simulink model "HDL_source"  (R2019a)
settings: Solver=FixedStepDiscrete  StartTime=0.0  StopTime=0.1  RelTol=1e-3
PreLoadFcn:
  | load('visionhdlLaneDetectionInit.mat');
  | 
  | %Birds-Eye View Parameters:
  | T_unreal = [-0.346719845290643,-3.45626583672944e-16,-2.42608110520569e-19;-1.76272742794994,-2.62399506819665,-0.00185184300876343;1283.14845282490,1569.57420684550,1];
  | shiftleft = single([-5,-5,-5,-5,-5,-5,-5,-5,-5,-5,   -5,-4,-2,-2,-2,-2,0,0,0,1,    1,2,3,4,5,6,7,10,11,13,     15,17,20,22,26,30,33,38,42,46]);
  | shiftright = single([-20,-20,-20,-20,-20,-20,-20,-20,-20,-20,    -20,-20,-20,-21,-22,-23,-24,-24,-24,-25,    -26,-27,-28,-29,-30,-32,-33,-35,-37,-39,    -41,-45,-46,-50,-53,-57,-61,-67,-72,-78]);
StartFcn:
  | warning('off','Coder:MATLAB:polyfit_RepeatedPointsOrRescale');
  | warning('off','Coder:MATLAB:rankDeficientMatrix');
StopFcn:
  | warning('on','Coder:MATLAB:polyfit_RepeatedPointsOrRescale');
  | warning('on','Coder:MATLAB:rankDeficientMatrix');
undefined symbols (not defined in the file): gray, h1, imresize, Rec, SDTV
libraries: simulink x31, hdlsllib x19, visionhdlutilities x6, visionhdlstatistics x4, visiongeotforms x3, visionhdlio x2, visiontextngfix x2, visionhdlconversions x1, visionhdlgeotforms x1, visionhdlfilter x1, dspvision x1, visionsinks x1
(part 1 of 3)
Description:
  | Lane Detection
  | Detect lanes from streaming video.
settings Model: DataTypeOverride=Off  Creator=The MathWorks, Inc.  LastModifiedBy=timo.straessle
settings DataIOCC: SaveOutput=off  SaveTime=off  ReturnWorkspaceOutputs=off
settings OptimizationCC: BlockReduction=off  ConditionallyExecuteInputs=off  DefaultParameterBehavior=Inlined  EfficientMapNaN2IntZero=off
settings DebuggingCC: AlgebraicLoopMsg=error  SingleTaskRateTransMsg=error  ParameterPrecisionLossMsg=none  StrictBusMsg=ErrorOnBusTreatedAsVector  ArithmeticOperatorsInVariantConditions=warning
settings HardwareCC: ProdBitPerPointer=32  ProdBitPerSizeT=32  ProdBitPerPtrDiffT=32  ProdLargestAtomicFloat=None  ProdIntDivRoundTo=Undefined  ProdEndianess=Unspecified  ProdWordSize=32  ProdHWDeviceType=ASIC/FPGA->ASIC/FPGA  TargetBitPerPointer=64  TargetBitPerSizeT=64  TargetBitPerPtrDiffT=64  TargetLongLongMode=on  TargetIntDivRoundTo=Zero  TargetEndianess=LittleEndian  TargetWordSize=64  TargetHWDeviceType=MATLAB Host  ProdEqTarget=off
settings SFSimCC: SimUseLocalCustomCode=off
settings RTWCC: TLCOptions=-axpcCPUClockPoll=0
settings CodeAppCC: MaxIdLength=128
settings GRTTargetCC: TargetLangStandard=C89/C90 (ANSI)  CombineOutputUpdateFcns=off  GRTInterface=on
settings ConfigComp: CovMetricSettings=dsw  CovHtmlReporting=on  CovSaveCumulativeToWorkspaceVar=on  CovSaveSingleToWorkspaceVar=on  CovShowResultsExplorer=off  CovExternalEMLEnable=off

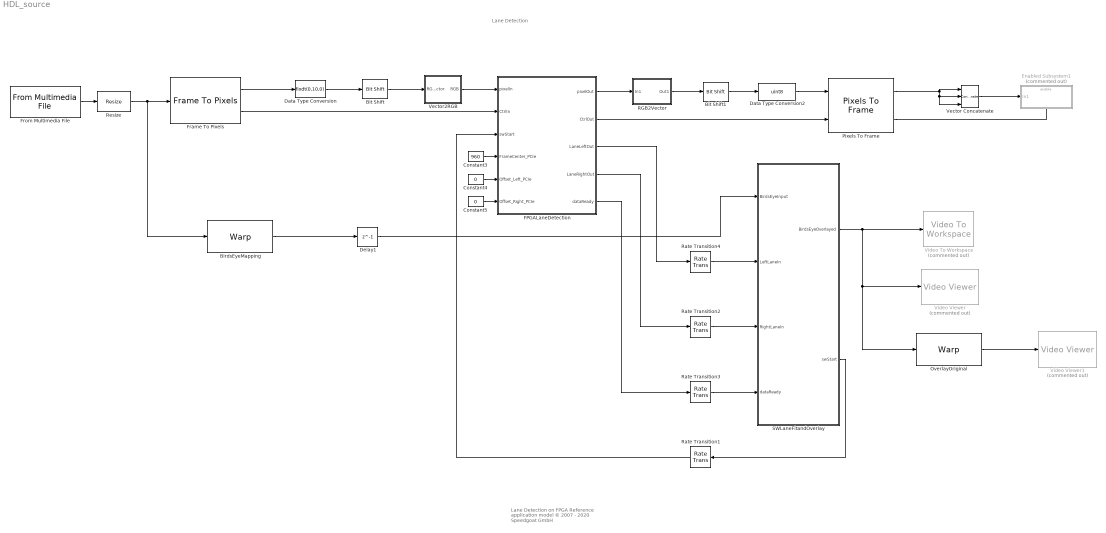
== system HDL_source ==
  note: Lane Detection
  note: Lane Detection on FPGA
      |
      | Reference application model
      | © 2007 - 2020 Speedgoat GmbH
  BirdsEyeMapping : visiongeotforms/Warp  TransformMatrixSource=Custom  TransformMatrix=T_unreal  InterpolationMethod=Bilinear  BackgroundFillValue=0  OutputImagePositionSource=Custom  OutputImagePosition=[ 1, 1, 1920, 1080 ]  ROIInputPort=off  ROIValidityOutputPort=off  SimulateUsing=Code generation
      settings: SourceProductName=Computer Vision Toolbox  SourceProductBaseCode=VP
  Bit Shift : hdlsllib/Logic and Bit Operations/Bit Shift  mode=Shift Left Logical  N=2
      settings: SourceProductName=Simulink
  Bit Shift1 : hdlsllib/Logic and Bit Operations/Bit Shift  mode=Shift Right Logical  N=2
      settings: SourceProductName=Simulink
  Constant3 : Constant  Value=960  OutDataTypeStr=fixdt(1,12,2^0,0)  SampleTime=-1
  Constant4 : Constant  Value=0  OutDataTypeStr=Inherit: Inherit via back propagation  SampleTime=-1
  Constant5 : Constant  Value=0  OutDataTypeStr=Inherit: Inherit via back propagation  SampleTime=-1
  Data Type Conversion : DataTypeConversion  OutDataTypeStr=fixdt(0,10,0)  RndMeth=Nearest
  Data Type Conversion2 : DataTypeConversion  OutDataTypeStr=uint8
  Delay1 : Delay  DelayLength=1
  Enabled Subsystem1 : Subsystem  Commented=on  TreatAsAtomicUnit=on
  FPGALaneDetection : Subsystem
  Frame To Pixels : visionhdlio/Frame To Pixels  NumComponents=3  VideoFormat=1080p  ActivePixelsPerLine=160  ActiveVideoLines=160  TotalPixelsPerLine=400  TotalVideoLines=400  StartingActiveLine=6  FrontPorch=120  SampleTime=0
      settings: SourceProductName=Vision HDL Toolbox  SourceProductBaseCode=VT
  From Multimedia File : dspvision/From Multimedia File  inputFilename=unreal.mp4  readRange=[1 Inf]  loop=on  numPlays=inf  outputStreams=Video only  videoDataType=uint8  audioDataType=int16  inheritSampleTime=off  userDefinedSampleTime=1/60  noAudioOutput=off  isIntensityVideo=off  fourcc=RGB  colorVideoFormat=One multidimensional signal  outputEOF=off  dataOrg=Column-major  audioFrameSize=1024  computeAudioFrameSize=off  outSamplingMode=Sample based
      settings: SourceProductName=DSP System Toolbox  SourceProductBaseCode=DS
  OverlayOriginal : visiongeotforms/Warp  TransformMatrixSource=Custom  TransformMatrix=inv(T_unreal)  InterpolationMethod=Bilinear  BackgroundFillValue=0  OutputImagePositionSource=Custom  OutputImagePosition=[ 1, 1, 1920, 1080 ]  ROIInputPort=off  ROIValidityOutputPort=off  SimulateUsing=Code generation
      settings: SourceProductName=Computer Vision Toolbox  SourceProductBaseCode=VP
  Pixels To Frame : visionhdlio/Pixels To Frame  NumComponents=1  VideoFormat=1080p  ActivePixelsPerLine=720  ActiveVideoLines=540  TotalPixelsPerLine=2200  TotalVideoLines=1125
      settings: SourceProductName=Vision HDL Toolbox  SourceProductBaseCode=VT
  "RGB2Vector " : Subsystem
  Rate Transition{1..4} (4 alike) : RateTransition  Deterministic=off
  Resize : visiongeotforms/Resize  specify=Number of output rows and preserve aspect ratio  rfactor=[200 150]  outCols=25  outRows=1080  outRowsCols=[25 35]  interp_method=Bilinear  antialias=on  useROI=off  roiFlag=off  roundingMode=Nearest  overflowMode=on  prodOutputMode=Binary point scaling  prodOutputWordLength=32  prodOutputFracLength=10  prodOutputSlope=2^-10  accumSlope=2^-10  outputSlope=2^-10
      settings: SourceProductName=Computer Vision Toolbox  SourceProductBaseCode=VP
  SWLaneFitandOverlay : Subsystem
  Vector Concatenate : Concatenate  NumInputs=3  Mode=Multidimensional array  ConcatenateDimension=3
  Vector2RGB : Subsystem
  Video To Workspace : visionsinks/Video To Workspace  Commented=on  VariableName=vout  NumInputs=1  DataLimit=10  DecimationFactor=1  LogFi=off  InPortLabels=R|G|B
      settings: SourceProductName=Computer Vision Toolbox  SourceProductBaseCode=VP
  Video Viewer : VideoViewer  Commented=on  colormapValue=gray(256)  FigPos=[1223 878 558 588]
  Video Viewer1 : VideoViewer  Commented=on  colormapValue=gray(256)  FigPos=[1085 664 697 473]
  wires:
  Data Type Conversion/1 -> Bit Shift/1
  Vector2RGB/1(RGB) -> FPGALaneDetection/1(pixelIn)
  Frame To Pixels/2 -> FPGALaneDetection/2(CtrlIn)
  Rate Transition1/1 -> FPGALaneDetection/3(swStart)
  FPGALaneDetection/2(CtrlOut) -> Pixels To Frame/2
  Pixels To Frame/2 -> Enabled Subsystem1/Enable
  Frame To Pixels/1 -> Data Type Conversion/1
  Bit Shift/1 -> Vector2RGB/1(RGBVector)
  OverlayOriginal/1 -> Video Viewer1/1
  Delay1/1 -> SWLaneFitandOverlay/1(BirdsEyeInput)
  FPGALaneDetection/4(LaneRightOut) -> Rate Transition2/1
  FPGALaneDetection/5(dataReady) -> Rate Transition3/1
  Rate Transition3/1 -> SWLaneFitandOverlay/4(dataReady)
  SWLaneFitandOverlay/1(BirdsEyeOverlayed) -> Video Viewer/1, OverlayOriginal/1, Video To Workspace/1
  FPGALaneDetection/3(LaneLeftOut) -> Rate Transition4/1
  SWLaneFitandOverlay/2(swStart) -> Rate Transition1/1
  BirdsEyeMapping/1 -> Delay1/1
  FPGALaneDetection/1(pixelOut) -> "RGB2Vector "/1(In1)
  Pixels To Frame/1 -> Vector Concatenate/2, Vector Concatenate/3, Vector Concatenate/1
  Vector Concatenate/1 -> Enabled Subsystem1/1(In1)
  Constant3/1 -> FPGALaneDetection/4(FrameCenter_PCIe)
  Constant4/1 -> FPGALaneDetection/5(Offset_Left_PCIe)
  Constant5/1 -> FPGALaneDetection/6(Offset_Right_PCIe)
  "RGB2Vector "/1(Out1) -> Bit Shift1/1
  Bit Shift1/1 -> Data Type Conversion2/1
  Data Type Conversion2/1 -> Pixels To Frame/1
  From Multimedia File/1 -> Resize/1
  Rate Transition4/1 -> SWLaneFitandOverlay/2(LeftLaneIn)
  Rate Transition2/1 -> SWLaneFitandOverlay/3(RightLaneIn)
  Resize/1 -> BirdsEyeMapping/1, Frame To Pixels/1

== system HDL_source/Enabled Subsystem1 ==
  In1 : Inport
  Enable : EnablePort
  To Workspace : ToWorkspace  Commented=on  VariableName=imgmat  SaveFormat=Timeseries  SampleTime=-1
  Video Viewer : VideoViewer  colormapValue=gray(256)  FigPos=[100 917 1087 696]
  wires:
  In1/1 -> To Workspace/1, Video Viewer/1

== system HDL_source/FPGALaneDetection ==
  pixelIn : Inport
  CtrlIn : Inport  Port=2
  swStart : Inport  Port=3
  FrameCenter_PCIe : Inport  Port=4
  Offset_Left_PCIe : Inport  Port=5
  Offset_Right_PCIe : Inport  Port=6
  Bit Concat : hdlsllib/Logic and Bit Operations/Bit Concat  numInputs=3
      settings: SourceProductName=Simulink
  Bit Shift1 : hdlsllib/Logic and Bit Operations/Bit Shift  mode=Shift Left Logical  N=2
      settings: SourceProductName=Simulink
  Bit Slice : hdlsllib/Logic and Bit Operations/Bit Slice  lidx=9  ridx=2
      settings: SourceProductName=Simulink  SourceProductBaseCode=SL
  Color Space Converter : visionhdlconversions/Color Space Converter  Conversion=RGB to intensity  ConversionStandard=Rec. 601 (SDTV)  ScanningStandard=1250/50/2:1  SimulateUsing=Code generation
      settings: SourceProductName=Vision HDL Toolbox  SourceProductBaseCode=VT
  Data Type Conversion1 : DataTypeConversion  OutDataTypeStr=fixdt(0,10,0)  RndMeth=Nearest
  Lane Detection Algorithm : Subsystem  TreatAsAtomicUnit=on
  "RGB2Vector " : Subsystem
  pixelOut : Outport
  CtrlOut : Outport  Port=2
  LaneLeftOut : Outport  Port=3
  LaneRightOut : Outport  Port=4
  dataReady : Outport  Port=5
  wires:
  swStart/1 -> Lane Detection Algorithm/3(swStart)
  Lane Detection Algorithm/3(LeftLane) -> LaneLeftOut/1
  Lane Detection Algorithm/4(RightLane) -> LaneRightOut/1
  Lane Detection Algorithm/5(dataReady) -> dataReady/1
  FrameCenter_PCIe/1 -> Lane Detection Algorithm/4(FrameCenter_PCIe)
  Offset_Left_PCIe/1 -> Lane Detection Algorithm/5(Offset_Left_PCIe)
  Offset_Right_PCIe/1 -> Lane Detection Algorithm/6(Offset_Right_PCIe)
  pixelIn/1 -> "RGB2Vector "/1(In1)
  "RGB2Vector "/1(Out1) -> Bit Slice/1
  CtrlIn/1 -> Color Space Converter/2
  Color Space Converter/1 -> Lane Detection Algorithm/1(YIn)
  Color Space Converter/2 -> Lane Detection Algorithm/2(CtrlIn)
  Lane Detection Algorithm/2(CtrlOut) -> CtrlOut/1
  Data Type Conversion1/1 -> Bit Shift1/1
  Bit Slice/1 -> Color Space Converter/1
  Bit Concat/1 -> pixelOut/1
  Lane Detection Algorithm/1(YOut) -> Data Type Conversion1/1
  Bit Shift1/1 -> Bit Concat/3, Bit Concat/2, Bit Concat/1

== system HDL_source/RGB2Vector  ==
  In1 : Inport
  Bit Slice2 : hdlsllib/Logic and Bit Operations/Bit Slice  lidx=9  ridx=0
      settings: SourceProductName=Simulink  SourceProductBaseCode=SL
  Out1 : Outport  VectorParamsAs1DForOutWhenUnconnected=on
  wires:
  In1/1 -> Bit Slice2/1
  Bit Slice2/1 -> Out1/1

== system HDL_source/SWLaneFitandOverlay ==
  BirdsEyeInput : Inport
  LeftLaneIn : Inport  Port=2
  RightLaneIn : Inport  Port=3
  dataReady : Inport  Port=4
  Data Type Conversion : DataTypeConversion  OutDataTypeStr=single
  Data Type Conversion1 : DataTypeConversion  OutDataTypeStr=single
  Driver : MATLAB Function  TreatAsAtomicUnit=on
  FitLanesAndOverlay : Subsystem
  Rate Transition1 : RateTransition  Deterministic=off  OutPortSampleTime=1/180
  Rate Transition2 : RateTransition  OutPortSampleTimeOpt=Inherit  OutPortSampleTime=1/60
  Signal Specification : SignalSpecification  OutDataTypeStr=boolean  Dimensions=1
  Signal Specification1 : SignalSpecification  OutDataTypeStr=boolean  Dimensions=1
  Signal Specification2 : SignalSpecification  SampleTime=1/180
  Signal Specification3 : SignalSpecification  SampleTime=1/180
  Signal Specification4 : SignalSpecification  SampleTime=1/720
  BirdsEyeOverlayed : Outport
  swStart : Outport  Port=2
  wires:
  BirdsEyeInput/1 -> FitLanesAndOverlay/1(BirdsEyeInput)
  FitLanesAndOverlay/1(OverlayOutput) -> BirdsEyeOverlayed/1
  LeftLaneIn/1 -> Signal Specification2/1
  RightLaneIn/1 -> Signal Specification3/1
  Signal Specification4/1 -> Driver/1(dataReady)
  Signal Specification/1 -> swStart/1
  Rate Transition1/1 -> FitLanesAndOverlay/Enable, Rate Transition2/1
  Rate Transition2/1 -> Signal Specification1/1
  Driver/2(process) -> Rate Transition1/1
  Signal Specification1/1 -> Driver/2(swDone)
  Driver/1(swStart) -> Signal Specification/1
  dataReady/1 -> Signal Specification4/1
  Signal Specification2/1 -> Data Type Conversion/1
  Signal Specification3/1 -> Data Type Conversion1/1
  Data Type Conversion/1 -> FitLanesAndOverlay/2(LeftLane)
  Data Type Conversion1/1 -> FitLanesAndOverlay/3(RightLane)

== system HDL_source/Vector2RGB ==
  RGBVector : Inport
  Bit Concat : hdlsllib/Logic and Bit Operations/Bit Concat  numInputs=3
      settings: SourceProductName=Simulink
  Demux : Demux  Outputs=3
  RGB : Outport  VectorParamsAs1DForOutWhenUnconnected=on
  wires:
  RGBVector/1 -> Demux/1
  Demux/1 -> Bit Concat/1
  Demux/2 -> Bit Concat/2
  Demux/3 -> Bit Concat/3
  Bit Concat/1 -> RGB/1

== system HDL_source/FPGALaneDetection/Lane Detection Algorithm ==
  YIn : Inport
  CtrlIn : Inport  Port=2
  swStart : Inport  Port=3
  FrameCenter_PCIe : Inport  Port=4
  Offset_Left_PCIe : Inport  Port=5
  Offset_Right_PCIe : Inport  Port=6
  Birds-Eye View : visionhdlgeotforms/Birds-Eye View  HomographyMatrix=T_unreal  MaxBufferSize=400000  MaxSourceLinesBuffered=200  BirdsEyeActivePixels=1920  BirdsEyeActiveLines=1080  SimulateUsing=Code generation
      settings: SourceProductName=Vision HDL Toolbox  SourceProductBaseCode=VT
  ComputeEgoLanes1 : Subsystem
  CtrlInterface1 : MATLAB Function  TreatAsAtomicUnit=on
  LaneDetection1 : Subsystem
  Signal Specification3 : SignalSpecification  Dimensions=[40 1]
  Signal Specification4 : SignalSpecification  Dimensions=[40 1]
  Signal Specification5 : SignalSpecification  OutDataTypeStr=boolean
  YOut : Outport
  CtrlOut : Outport  Port=2
  LeftLane : Outport  Port=3
  RightLane : Outport  Port=4
  dataReady : Outport  Port=5
  wires:
  Birds-Eye View/2 -> CtrlOut/1, LaneDetection1/2(ctrlIn)
  FrameCenter_PCIe/1 -> ComputeEgoLanes1/10(Frame_Center_PCIe)
  Offset_Left_PCIe/1 -> ComputeEgoLanes1/11(Offset_Left_PCIe)
  Offset_Right_PCIe/1 -> ComputeEgoLanes1/12(Offset_Right_PCIe)
  CtrlInterface1/1(LaneLeftout) -> Signal Specification3/1
  LaneDetection1/5(lane4) -> ComputeEgoLanes1/5(lane4In)
  ComputeEgoLanes1/4(start) -> CtrlInterface1/4(hwStart)
  ComputeEgoLanes1/5(done) -> CtrlInterface1/5(hwDone)
  LaneDetection1/8(lane7) -> ComputeEgoLanes1/8(lane7In)
  swStart/1 -> CtrlInterface1/6(swStart)
  LaneDetection1/7(lane6) -> ComputeEgoLanes1/7(lane6In)
  LaneDetection1/6(lane5) -> ComputeEgoLanes1/6(lane5In)
  ComputeEgoLanes1/3(enable) -> CtrlInterface1/3(enable)
  LaneDetection1/3(lane2) -> ComputeEgoLanes1/3(lane2In)
  LaneDetection1/1(enable) -> ComputeEgoLanes1/1(laneCapture)
  ComputeEgoLanes1/2(LaneRight) -> CtrlInterface1/2(LaneRightin)
  LaneDetection1/9(frameStart) -> ComputeEgoLanes1/9(frameStart)
  Signal Specification4/1 -> RightLane/1
  Signal Specification5/1 -> dataReady/1
  Signal Specification3/1 -> LeftLane/1
  CtrlInterface1/3(dataReady) -> Signal Specification5/1
  CtrlInterface1/2(LaneRightout) -> Signal Specification4/1
  ComputeEgoLanes1/1(LaneLeft) -> CtrlInterface1/1(LaneLeftin)
  LaneDetection1/4(lane3) -> ComputeEgoLanes1/4(lane3In)
  LaneDetection1/2(lane1) -> ComputeEgoLanes1/2(lane1In)
  Birds-Eye View/1 -> YOut/1, LaneDetection1/1(pixelIn)
  YIn/1 -> Birds-Eye View/1
  CtrlIn/1 -> Birds-Eye View/2

== system HDL_source/FPGALaneDetection/RGB2Vector  ==
  In1 : Inport
  Bit Slice : hdlsllib/Logic and Bit Operations/Bit Slice  lidx=29  ridx=20
      settings: SourceProductName=Simulink  SourceProductBaseCode=SL
  Bit Slice1 : hdlsllib/Logic and Bit Operations/Bit Slice  lidx=19  ridx=10
      settings: SourceProductName=Simulink  SourceProductBaseCode=SL
  Bit Slice2 : hdlsllib/Logic and Bit Operations/Bit Slice  lidx=9  ridx=0
      settings: SourceProductName=Simulink  SourceProductBaseCode=SL
  Mux : Mux  Inputs=3
  Transpose : Math  Operator=transpose  RndMeth=Zero  SaturateOnIntegerOverflow=on
  Out1 : Outport  VectorParamsAs1DForOutWhenUnconnected=on
  wires:
  In1/1 -> Bit Slice2/1, Bit Slice1/1, Bit Slice/1
  Bit Slice/1 -> Mux/1
  Bit Slice1/1 -> Mux/2
  Bit Slice2/1 -> Mux/3
  Mux/1 -> Transpose/1
  Transpose/1 -> Out1/1

== system HDL_source/SWLaneFitandOverlay/FitLanesAndOverlay ==
  BirdsEyeInput : Inport
  LeftLane : Inport  Port=2
  RightLane : Inport  Port=3
  Enable : EnablePort
  Add : Sum
  Add1 : Sum
  Constant : Constant  Value=shiftleft
  Constant1 : Constant  Value=shiftright
  FitLanes : Subsystem
  Index : Constant  Value=[1:1:40]'*27  VectorParams1D=off  OutDataTypeStr=single  SampleTime=-1
  OverlayLaneMarkings : Subsystem
  Rate Transition{,1..3} (4 alike) : RateTransition  OutPortSampleTime=1/60
  Vector Concatenate : Concatenate  Mode=Multidimensional array  ConcatenateDimension=2
  Vector Concatenate1 : Concatenate  Mode=Multidimensional array  ConcatenateDimension=2
  OverlayOutput : Outport
  wires:
  FitLanes/2(RightPolynomial) -> Rate Transition1/1
  FitLanes/1(LeftPolynomial) -> Rate Transition/1
  OverlayLaneMarkings/1(ImOut) -> OverlayOutput/1
  LeftLane/1 -> Add/2
  Rate Transition/1 -> OverlayLaneMarkings/4(LeftPolynomial)
  Rate Transition1/1 -> OverlayLaneMarkings/5(RightPolynomial)
  Vector Concatenate1/1 -> Rate Transition3/1, FitLanes/2(RightLaneCoords)
  Vector Concatenate/1 -> FitLanes/1(LeftLaneCoords), Rate Transition2/1
  BirdsEyeInput/1 -> OverlayLaneMarkings/1(ImIn)
  RightLane/1 -> Add1/2
  Index/1 -> Vector Concatenate/2, Vector Concatenate1/2
  Rate Transition2/1 -> OverlayLaneMarkings/2(LeftLaneCoords)
  Rate Transition3/1 -> OverlayLaneMarkings/3(RightLaneCoords)
  Constant/1 -> Add/1
  Add/1 -> Vector Concatenate/1
  Constant1/1 -> Add1/1
  Add1/1 -> Vector Concatenate1/1

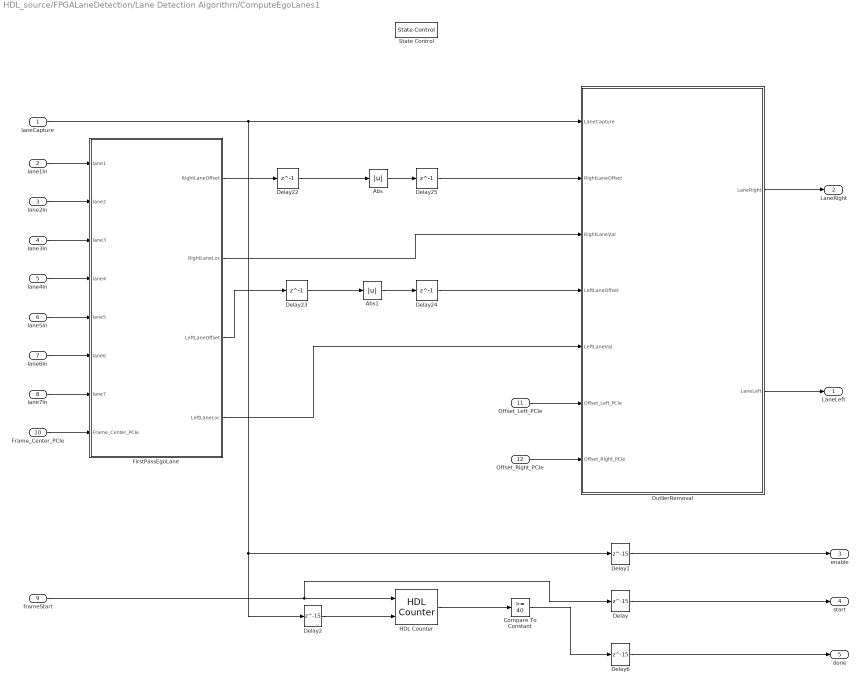
== system HDL_source/FPGALaneDetection/Lane Detection Algorithm/ComputeEgoLanes1 ==
  laneCapture : Inport
  lane1In : Inport  Port=2
  lane2In : Inport  Port=3
  lane3In : Inport  Port=4
  lane4In : Inport  Port=5
  lane5In : Inport  Port=6
  lane6In : Inport  Port=7
  lane7In : Inport  Port=8
  frameStart : Inport  Port=9
  Frame_Center_PCIe : Inport  Port=10
  Offset_Left_PCIe : Inport  Port=11
  Offset_Right_PCIe : Inport  Port=12
  Abs : Abs
  Abs1 : Abs
  Compare To Constant : simulink/Logic and Bit Operations/Compare To Constant  relop=>=  const=40  OutDataTypeStr=boolean
  Delay{,1..2,6} (4 alike) : Delay  DelayLength=15
  Delay{22..25} (4 alike) : Delay  DelayLength=1
  FirstPassEgoLane : Subsystem
  HDL Counter : hdlsllib/Sources/HDL Counter  CountType=Free running  CountInit=0  CountStep=1  CountMax=40  CountFromType=Initial value  CountFrom=0  CountResetPort=on  CountLoadPort=off  CountEnbPort=on  CountDirPort=off  CountDataType=Unsigned  CountWordLen=6  CountFracLen=0  CountSampTime=1
      settings: SourceProductName=Simulink
  OutlierRemoval : Subsystem
  State Control : StateControl  StateControl=Synchronous
  LaneLeft : Outport
  LaneRight : Outport  Port=2
  enable : Outport  Port=3
  start : Outport  Port=4
  done : Outport  Port=5
  wires:
  laneCapture/1 -> Delay1/1, Delay2/1, OutlierRemoval/1(LaneCapture)
  Abs/1 -> Delay25/1
  Abs1/1 -> Delay24/1
  lane1In/1 -> FirstPassEgoLane/1(lane1)
  lane2In/1 -> FirstPassEgoLane/2(lane2)
  lane3In/1 -> FirstPassEgoLane/3(lane3)
  lane4In/1 -> FirstPassEgoLane/4(lane4)
  lane5In/1 -> FirstPassEgoLane/5(lane5)
  lane6In/1 -> FirstPassEgoLane/6(lane6)
  lane7In/1 -> FirstPassEgoLane/7(lane7)
  FirstPassEgoLane/1(RightLaneOffset) -> Delay22/1
  FirstPassEgoLane/3(LeftLaneOffset) -> Delay23/1
  Delay22/1 -> Abs/1
  Delay23/1 -> Abs1/1
  Delay25/1 -> OutlierRemoval/2(RightLaneOffset)
  FirstPassEgoLane/2(RightLaneLoc) -> OutlierRemoval/3(RightLaneVal)
  FirstPassEgoLane/4("LeftLaneLoc ") -> OutlierRemoval/5(LeftLaneVal)
  Delay24/1 -> OutlierRemoval/4(LeftLaneOffset)
  Delay/1 -> start/1
  Delay6/1 -> done/1
  Delay1/1 -> enable/1
  OutlierRemoval/1(LaneRight) -> LaneRight/1
  OutlierRemoval/2(LaneLeft) -> LaneLeft/1
  HDL Counter/1 -> Compare To Constant/1
  frameStart/1 -> Delay/1, HDL Counter/1
  Compare To Constant/1 -> Delay6/1
  Delay2/1 -> HDL Counter/2
  Frame_Center_PCIe/1 -> FirstPassEgoLane/8(Frame_Center_PCIe)
  Offset_Left_PCIe/1 -> OutlierRemoval/6(Offset_Left_PCIe)
  Offset_Right_PCIe/1 -> OutlierRemoval/7(Offset_Right_PCIe)

== system HDL_source/FPGALaneDetection/Lane Detection Algorithm/LaneDetection1 ==
  pixelIn : Inport
  ctrlIn : Inport  Port=2
  LaneCandidateGeneration : Subsystem
  State Control : StateControl  StateControl=Synchronous
  VerticallyOrientatedFilter : visionhdlfilter/Image Filter  CoefficientsSource=Property  Coefficients=imresize(h1, 2.25)/(2.25^2)  PaddingMethod=Symmetric  PaddingValue=0  LineBufferSize=2048  SimulateUsing=Code generation  roundingMode=Round  overflowMode=on  CoeffDataTypeStr=fixdt(1,24,15)  CoeffMin=[]  CoeffMax=[]  OutputDataTypeStr=fixdt(1,24,15)  OutputMin=[]  OutputMax=[]
      settings: SourceProductName=Vision HDL Toolbox  SourceProductBaseCode=VT
  enable : Outport
  lane1 : Outport  Port=2
  lane2 : Outport  Port=3
  lane3 : Outport  Port=4
  lane4 : Outport  Port=5
  lane5 : Outport  Port=6
  lane6 : Outport  Port=7
  lane7 : Outport  Port=8
  frameStart : Outport  Port=9
  wires:
  VerticallyOrientatedFilter/2 -> LaneCandidateGeneration/2(crtlIn)
  VerticallyOrientatedFilter/1 -> LaneCandidateGeneration/1(pixelIn)
  LaneCandidateGeneration/6(lane6) -> lane6/1
  ctrlIn/1 -> VerticallyOrientatedFilter/2
  LaneCandidateGeneration/4(lane4) -> lane4/1
  LaneCandidateGeneration/3(lane3) -> lane3/1
  LaneCandidateGeneration/7(lane7) -> lane7/1
  LaneCandidateGeneration/2(lane2) -> lane2/1
  pixelIn/1 -> VerticallyOrientatedFilter/1
  LaneCandidateGeneration/8(laneCapture) -> enable/1
  LaneCandidateGeneration/5(lane5) -> lane5/1
  LaneCandidateGeneration/1(lane1) -> lane1/1
  LaneCandidateGeneration/9(frameStart) -> frameStart/1

== system HDL_source/SWLaneFitandOverlay/FitLanesAndOverlay/FitLanes ==
  LeftLaneCoords : Inport
  RightLaneCoords : Inport  Port=2
  FitLeftPolyLane : MATLAB Function  TreatAsAtomicUnit=on
  FitRightPolyLane : MATLAB Function  TreatAsAtomicUnit=on
  LeftPolynomial : Outport
  RightPolynomial : Outport  Port=2
  wires:
  FitLeftPolyLane/1(P) -> LeftPolynomial/1
  FitRightPolyLane/1(P) -> RightPolynomial/1
  LeftLaneCoords/1 -> FitLeftPolyLane/1(laneCIn)
  RightLaneCoords/1 -> FitRightPolyLane/1(laneCIn)

== system HDL_source/SWLaneFitandOverlay/FitLanesAndOverlay/OverlayLaneMarkings ==
  ImIn : Inport
  LeftLaneCoords : Inport  Port=2
  RightLaneCoords : Inport  Port=3
  LeftPolynomial : Inport  Port=4
  RightPolynomial : Inport  Port=5
  Constant{,1..3} (4 alike) : Constant  Value=ones(40,1)*30  OutDataTypeStr=single  SampleTime=-1
  Constant4 : Constant  Value=[75 1 1845 1080]  OutDataTypeStr=uint32  SampleTime=-1
  Constant5 : Constant  Value=[75 1 1845 1080]  OutDataTypeStr=uint32  SampleTime=-1
  Data Type Conversion : DataTypeConversion  OutDataTypeStr=uint32
  Data Type Conversion1 : DataTypeConversion  OutDataTypeStr=uint32
  Draw Shapes : visiontextngfix/Draw Shapes  shape=Rectangles  fill=off  lineWidth=4  fillClrSource=Specify via dialog  display=User-specified value  intensity=200  color=[83, 219, 192]  opacity=0.6  viewport=Specify region of interest via port  antialiasing=off  inType=Obsolete  imagePorts=One multidimensional signal  roundingMode=Floor  overflowMode=off  memoryMode=Specify word length  memoryWordLength=16  prodOutputMode=Binary point scaling  prodOutputWordLength=32  prodOutputFracLength=14  prodOutputSlope=2^-14  accumSlope=2^-14  memoryFracLength=15
      settings: SourceProductName=Computer Vision Toolbox
  Draw Shapes1 : visiontextngfix/Draw Shapes  shape=Rectangles  fill=off  lineWidth=4  fillClrSource=Specify via dialog  display=User-specified value  intensity=200  color=[255, 26,0]  opacity=0.6  viewport=Specify region of interest via port  antialiasing=off  inType=Obsolete  imagePorts=One multidimensional signal  roundingMode=Floor  overflowMode=off  memoryMode=Specify word length  memoryWordLength=16  prodOutputMode=Binary point scaling  prodOutputWordLength=32  prodOutputFracLength=14  prodOutputSlope=2^-14  accumSlope=2^-14  memoryFracLength=15
      settings: SourceProductName=Computer Vision Toolbox
  DrawPolynomial : MATLAB Function  TreatAsAtomicUnit=on
  OverlayPolynomialLane1 : MATLAB Function  TreatAsAtomicUnit=on
  Vector Concatenate{,1..3} (4 alike) : Concatenate  Mode=Multidimensional array  ConcatenateDimension=2
  ImOut : Outport
  wires:
  OverlayPolynomialLane1/1(Im) -> DrawPolynomial/2("Im ")
  DrawPolynomial/1(Im) -> ImOut/1
  LeftPolynomial/1 -> OverlayPolynomialLane1/1(P1)
  RightPolynomial/1 -> DrawPolynomial/1(P1)
  Constant/1 -> Vector Concatenate/2
  LeftLaneCoords/1 -> Vector Concatenate/1
  Constant1/1 -> Vector Concatenate1/2
  Vector Concatenate/1 -> Vector Concatenate1/1
  ImIn/1 -> Draw Shapes1/1
  RightLaneCoords/1 -> Vector Concatenate2/1
  Vector Concatenate1/1 -> Data Type Conversion/1
  Data Type Conversion/1 -> Draw Shapes1/2
  Draw Shapes1/1 -> Draw Shapes/1
  Vector Concatenate3/1 -> Data Type Conversion1/1
  Vector Concatenate2/1 -> Vector Concatenate3/1
  Constant3/1 -> Vector Concatenate3/2
  Constant2/1 -> Vector Concatenate2/2
  Data Type Conversion1/1 -> Draw Shapes/2
  Draw Shapes/1 -> OverlayPolynomialLane1/2("Im ")
  Constant4/1 -> Draw Shapes1/3
  Constant5/1 -> Draw Shapes/3

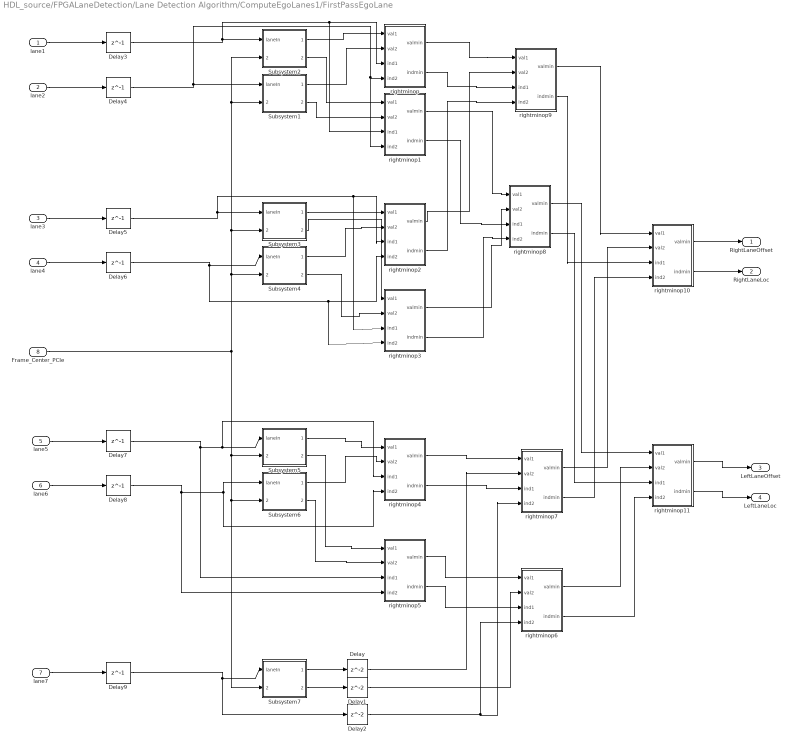
== system HDL_source/FPGALaneDetection/Lane Detection Algorithm/ComputeEgoLanes1/FirstPassEgoLane ==
  lane1 : Inport
  lane2 : Inport  Port=2
  lane3 : Inport  Port=3
  lane4 : Inport  Port=4
  lane5 : Inport  Port=5
  lane6 : Inport  Port=6
  lane7 : Inport  Port=7
  Frame_Center_PCIe : Inport  Port=8
  Delay : Delay
  Delay1 : Delay
  Delay2 : Delay
  Delay{3..9} (7 alike) : Delay  DelayLength=1
  Subsystem1 : Subsystem
  Subsystem2 : Subsystem
  Subsystem3 : Subsystem
  Subsystem4 : Subsystem
  Subsystem5 : Subsystem
  Subsystem6 : Subsystem
  Subsystem7 : Subsystem
  rightminop : Subsystem
  rightminop1 : Subsystem
  rightminop10 : Subsystem
  rightminop11 : Subsystem
  rightminop2 : Subsystem
  rightminop3 : Subsystem
  rightminop4 : Subsystem
  rightminop5 : Subsystem
  rightminop6 : Subsystem
  rightminop7 : Subsystem
  rightminop8 : Subsystem
  rightminop9 : Subsystem
  RightLaneOffset : Outport
  RightLaneLoc : Outport  Port=2
  LeftLaneOffset : Outport  Port=3
  "LeftLaneLoc " : Outport  Port=4
  wires:
  Subsystem7/2(LeftLaneVal) -> Delay1/1
  rightminop7/1(valmin) -> rightminop10/2(val2)
  rightminop9/2(indmin) -> rightminop10/3(ind1)
  rightminop3/2(indmin) -> rightminop8/4(ind2)
  rightminop7/2(indmin) -> rightminop10/4(ind2)
  Subsystem5/2(LeftLaneVal) -> rightminop5/1(val1)
  rightminop8/1(valmin) -> rightminop11/1(val1)
  Subsystem2/1(RightLaneVal) -> rightminop/1(val1)
  rightminop4/2(indmin) -> rightminop7/3(ind1)
  rightminop6/2(indmin) -> rightminop11/4(ind2)
  Subsystem1/1(RightLaneVal) -> rightminop/2(val2)
  Subsystem7/1(RightLaneVal) -> Delay/1
  Subsystem4/1(RightLaneVal) -> rightminop2/2(val2)
  rightminop5/2(indmin) -> rightminop6/3(ind1)
  rightminop6/1(valmin) -> rightminop11/2(val2)
  lane3/1 -> Delay5/1
  rightminop9/1(valmin) -> rightminop10/1(val1)
  rightminop8/2(indmin) -> rightminop11/3(ind1)
  rightminop5/1(valmin) -> rightminop6/1(val1)
  lane7/1 -> Delay9/1
  rightminop1/1(valmin) -> rightminop8/1(val1)
  rightminop11/1(valmin) -> LeftLaneOffset/1
  rightminop11/2(indmin) -> "LeftLaneLoc "/1
  rightminop/1(valmin) -> rightminop9/1(val1)
  rightminop3/1(valmin) -> rightminop8/2(val2)
  rightminop2/1(valmin) -> rightminop9/2(val2)
  Subsystem4/2(LeftLaneVal) -> rightminop3/2(val2)
  rightminop2/2(indmin) -> rightminop9/4(ind2)
  Subsystem3/1(RightLaneVal) -> rightminop2/1(val1)
  rightminop10/1(valmin) -> RightLaneOffset/1
  lane5/1 -> Delay7/1
  lane2/1 -> Delay4/1
  Subsystem3/2(LeftLaneVal) -> rightminop3/1(val1)
  rightminop10/2(indmin) -> RightLaneLoc/1
  Subsystem2/2(LeftLaneVal) -> rightminop1/1(val1)
  lane6/1 -> Delay8/1
  Subsystem6/1(RightLaneVal) -> rightminop4/2(val2)
  lane4/1 -> Delay6/1
  rightminop1/2(indmin) -> rightminop8/3(ind1)
  Subsystem5/1(RightLaneVal) -> rightminop4/1(val1)
  Subsystem6/2(LeftLaneVal) -> rightminop5/2(val2)
  rightminop/2(indmin) -> rightminop9/3(ind1)
  Subsystem1/2(LeftLaneVal) -> rightminop1/2(val2)
  rightminop4/1(valmin) -> rightminop7/1(val1)
  lane1/1 -> Delay3/1
  Delay/1 -> rightminop7/2(val2)
  Delay1/1 -> rightminop6/2(val2)
  Delay2/1 -> rightminop7/4(ind2), rightminop6/4(ind2)
  Delay3/1 -> Subsystem2/1(laneIn), rightminop1/3(ind1), rightminop/3(ind1)
  Delay4/1 -> Subsystem1/1(laneIn), rightminop1/4(ind2), rightminop/4(ind2)
  Delay5/1 -> Subsystem3/1(laneIn), rightminop3/3(ind1), rightminop2/3(ind1)
  Delay6/1 -> rightminop3/4(ind2), rightminop2/4(ind2), Subsystem4/1(laneIn)
  Delay7/1 -> rightminop5/3(ind1), rightminop4/3(ind1), Subsystem5/1(laneIn)
  Delay8/1 -> rightminop5/4(ind2), rightminop4/4(ind2), Subsystem6/1(laneIn)
  Delay9/1 -> Delay2/1, Subsystem7/1(laneIn)
  Frame_Center_PCIe/1 -> Subsystem7/2(Frame_Center_PCIe), Subsystem6/2(Frame_Center_PCIe), Subsystem5/2(Frame_Center_PCIe), Subsystem4/2(Frame_Center_PCIe), Subsystem2/2(Frame_Center_PCIe), Subsystem1/2(Frame_Center_PCIe), Subsystem3/2(Frame_Center_PCIe)

== system HDL_source/FPGALaneDetection/Lane Detection Algorithm/ComputeEgoLanes1/OutlierRemoval ==
  LaneCapture : Inport
  RightLaneOffset : Inport  Port=2
  RightLaneVal : Inport  Port=3
  LeftLaneOffset : Inport  Port=4
  LeftLaneVal : Inport  Port=5
  Offset_Left_PCIe : Inport  Port=6
  Offset_Right_PCIe : Inport  Port=7
  AverageLeftWidth : Subsystem
  AverageRightWidth : Subsystem
  Delay{2..5} (4 alike) : Delay  DelayLength=9
  RemoveOutlier : Subsystem
  RemoveOutlier1 : Subsystem
  Subtract : Sum  Inputs=+-
  Subtract1 : Sum  Inputs=+-
  UpdateLaneWidth : Subsystem
  LaneRight : Outport
  LaneLeft : Outport  Port=2
  wires:
  RightLaneVal/1 -> Delay3/1
  LeftLaneVal/1 -> Delay5/1
  Delay4/1 -> RemoveOutlier1/2(offsetVal)
  RemoveOutlier1/1(Inlier) -> LaneLeft/1
  LeftLaneOffset/1 -> AverageLeftWidth/1(data), Delay4/1, UpdateLaneWidth/4(LeftOffset)
  RightLaneOffset/1 -> AverageRightWidth/1(data), UpdateLaneWidth/2(RightOffset), Delay2/1
  Delay3/1 -> RemoveOutlier/1(laneVal)
  Delay2/1 -> RemoveOutlier/2(offsetVal)
  RemoveOutlier/1(Inlier) -> LaneRight/1
  Delay5/1 -> RemoveOutlier1/1(laneVal)
  UpdateLaneWidth/1(LaneWidth) -> RemoveOutlier1/3(width), RemoveOutlier/3(width)
  LaneCapture/1 -> UpdateLaneWidth/3(CaptureLane), AverageLeftWidth/2(Enable), AverageRightWidth/2(Enable)
  AverageRightWidth/1(average) -> Subtract/1
  Subtract/1 -> UpdateLaneWidth/1(rightwidth)
  Offset_Right_PCIe/1 -> Subtract/2
  AverageLeftWidth/1(average) -> Subtract1/1
  Subtract1/1 -> UpdateLaneWidth/5(leftwidth)
  Offset_Left_PCIe/1 -> Subtract1/2

== system HDL_source/FPGALaneDetection/Lane Detection Algorithm/LaneDetection1/LaneCandidateGeneration ==
  pixelIn : Inport
  crtlIn : Inport  Port=2
  Compare To Constant2 : simulink/Logic and Bit Operations/Compare To Constant  relop===  const=1920  OutDataTypeStr=boolean
  Delay : Delay  DelayLength=1
  Delay9 : Delay  DelayLength=1
  DelayBalance1 : Delay  DelayLength=22
  DelayBalance2 : Delay  DelayLength=22
  DelayBalance3 : Delay  DelayLength=22
  HistogramColumnCount : Subsystem
  OverlapandMultiply : Subsystem
  Pixel Control Bus Selector : BusSelector  OutputSignals=vStart
  StoreDominantLanes : Subsystem
  ZeroCrossingFilter : Subsystem
  lane1 : Outport
  lane2 : Outport  Port=2
  lane3 : Outport  Port=3
  lane4 : Outport  Port=4
  lane5 : Outport  Port=5
  lane6 : Outport  Port=6
  lane7 : Outport  Port=7
  laneCapture : Outport  Port=8
  frameStart : Outport  Port=9
  wires:
  HistogramColumnCount/4(NegativeHistogramCount) -> OverlapandMultiply/2(negHistCount)
  StoreDominantLanes/7(lane7) -> lane7/1
  StoreDominantLanes/6(lane6) -> lane6/1
  StoreDominantLanes/5(lane5) -> lane5/1
  StoreDominantLanes/4(lane4) -> lane4/1
  StoreDominantLanes/3(lane3) -> lane3/1
  StoreDominantLanes/2(lane2) -> lane2/1
  StoreDominantLanes/1(lane1) -> lane1/1
  Delay/1 -> StoreDominantLanes/3(PeakFIlterData)
  HistogramColumnCount/3(HistogramAddress) -> DelayBalance2/1
  HistogramColumnCount/1(PositiveHistogramCount) -> OverlapandMultiply/1(posHistCount)
  HistogramColumnCount/2(HistogramValid) -> DelayBalance1/1
  pixelIn/1 -> HistogramColumnCount/1(pixelIn)
  OverlapandMultiply/1(matchedHist) -> ZeroCrossingFilter/1(In1)
  Compare To Constant2/1 -> StoreDominantLanes/1(LaneCapture), laneCapture/1
  Delay9/1 -> StoreDominantLanes/2(PeakFIlterAddress), Compare To Constant2/1, StoreDominantLanes/4(laneAddress)
  crtlIn/1 -> Pixel Control Bus Selector/1, HistogramColumnCount/2(controlIn)
  DelayBalance1/1 -> ZeroCrossingFilter/2(In2)
  DelayBalance2/1 -> Delay9/1
  ZeroCrossingFilter/1(Out1) -> Delay/1
  Pixel Control Bus Selector/1 -> DelayBalance3/1  "<vStart>"
  DelayBalance3/1 -> frameStart/1

== system HDL_source/FPGALaneDetection/Lane Detection Algorithm/ComputeEgoLanes1/FirstPassEgoLane/Subsystem1 ==
  laneIn : Inport
  Frame_Center_PCIe : Inport  Port=2
  Abs1 : Abs
  Add : Sum  Inputs=+-  OutDataTypeStr=fixdt(1,12,0)
  Compare To Zero : simulink/Logic and Bit Operations/Compare To Zero  relop=<=  OutDataTypeStr=boolean
  Constant7 : Constant  Value=1000  OutDataTypeStr=fixdt(1,12,0)  SampleTime=-1
  Delay : Delay  DelayLength=1
  Delay1 : Delay  DelayLength=1
  Multiport Switch : MultiPortSwitch  DataPortOrder=Zero-based contiguous  Inputs=2  zeroidx=on
  Multiport Switch1 : MultiPortSwitch  DataPortOrder=Zero-based contiguous  Inputs=2  zeroidx=on
  RightLaneVal : Outport
  LeftLaneVal : Outport  Port=2
  wires:
  Delay1/1 -> LeftLaneVal/1
  Delay/1 -> RightLaneVal/1
  Abs1/1 -> Delay/1
  Multiport Switch1/1 -> Delay1/1
  Frame_Center_PCIe/1 -> Add/1
  Constant7/1 -> Multiport Switch1/3, Multiport Switch/2
  Multiport Switch/1 -> Abs1/1
  Add/1 -> Multiport Switch1/2, Multiport Switch/3, Compare To Zero/1
  laneIn/1 -> Add/2
  Compare To Zero/1 -> Multiport Switch1/1, Multiport Switch/1

== system HDL_source/FPGALaneDetection/Lane Detection Algorithm/ComputeEgoLanes1/FirstPassEgoLane/Subsystem2 ==
  laneIn : Inport
  Frame_Center_PCIe : Inport  Port=2
  Abs1 : Abs
  Add : Sum  Inputs=+-  OutDataTypeStr=fixdt(1,12,0)
  Compare To Zero : simulink/Logic and Bit Operations/Compare To Zero  relop=<=  OutDataTypeStr=boolean
  Constant7 : Constant  Value=1000  OutDataTypeStr=fixdt(1,12,0)  SampleTime=-1
  Delay : Delay  DelayLength=1
  Delay1 : Delay  DelayLength=1
  Multiport Switch : MultiPortSwitch  DataPortOrder=Zero-based contiguous  Inputs=2  zeroidx=on
  Multiport Switch1 : MultiPortSwitch  DataPortOrder=Zero-based contiguous  Inputs=2  zeroidx=on
  RightLaneVal : Outport
  LeftLaneVal : Outport  Port=2
  wires:
  Compare To Zero/1 -> Multiport Switch/1, Multiport Switch1/1
  Add/1 -> Compare To Zero/1, Multiport Switch/3, Multiport Switch1/2
  Multiport Switch/1 -> Abs1/1
  Constant7/1 -> Multiport Switch/2, Multiport Switch1/3
  Frame_Center_PCIe/1 -> Add/1
  Multiport Switch1/1 -> Delay1/1
  Abs1/1 -> Delay/1
  Delay/1 -> RightLaneVal/1
  Delay1/1 -> LeftLaneVal/1
  laneIn/1 -> Add/2

== system HDL_source/FPGALaneDetection/Lane Detection Algorithm/ComputeEgoLanes1/FirstPassEgoLane/Subsystem3 ==
  laneIn : Inport
  Frame_Center_PCIe : Inport  Port=2
  Abs1 : Abs
  Add : Sum  Inputs=+-  OutDataTypeStr=fixdt(1,12,0)
  Compare To Zero : simulink/Logic and Bit Operations/Compare To Zero  relop=<=  OutDataTypeStr=boolean
  Constant7 : Constant  Value=1000  OutDataTypeStr=fixdt(1,12,0)  SampleTime=-1
  Delay : Delay  DelayLength=1
  Delay1 : Delay  DelayLength=1
  Multiport Switch : MultiPortSwitch  DataPortOrder=Zero-based contiguous  Inputs=2  zeroidx=on
  Multiport Switch1 : MultiPortSwitch  DataPortOrder=Zero-based contiguous  Inputs=2  zeroidx=on
  RightLaneVal : Outport
  LeftLaneVal : Outport  Port=2
  wires:
  Compare To Zero/1 -> Multiport Switch/1, Multiport Switch1/1
  laneIn/1 -> Add/2
  Add/1 -> Compare To Zero/1, Multiport Switch/3, Multiport Switch1/2
  Multiport Switch/1 -> Abs1/1
  Constant7/1 -> Multiport Switch/2, Multiport Switch1/3
  Frame_Center_PCIe/1 -> Add/1
  Multiport Switch1/1 -> Delay1/1
  Abs1/1 -> Delay/1
  Delay/1 -> RightLaneVal/1
  Delay1/1 -> LeftLaneVal/1

== system HDL_source/FPGALaneDetection/Lane Detection Algorithm/ComputeEgoLanes1/FirstPassEgoLane/Subsystem4 ==
  laneIn : Inport
  Frame_Center_PCIe : Inport  Port=2
  Abs1 : Abs
  Add : Sum  Inputs=+-  OutDataTypeStr=fixdt(1,12,0)
  Compare To Zero : simulink/Logic and Bit Operations/Compare To Zero  relop=<=  OutDataTypeStr=boolean
  Constant7 : Constant  Value=1000  OutDataTypeStr=fixdt(1,12,0)  SampleTime=-1
  Delay : Delay  DelayLength=1
  Delay1 : Delay  DelayLength=1
  Multiport Switch : MultiPortSwitch  DataPortOrder=Zero-based contiguous  Inputs=2  zeroidx=on
  Multiport Switch1 : MultiPortSwitch  DataPortOrder=Zero-based contiguous  Inputs=2  zeroidx=on
  RightLaneVal : Outport
  LeftLaneVal : Outport  Port=2
  wires:
  Delay1/1 -> LeftLaneVal/1
  Delay/1 -> RightLaneVal/1
  Abs1/1 -> Delay/1
  Multiport Switch1/1 -> Delay1/1
  Frame_Center_PCIe/1 -> Add/1
  Constant7/1 -> Multiport Switch1/3, Multiport Switch/2
  Multiport Switch/1 -> Abs1/1
  Add/1 -> Multiport Switch1/2, Multiport Switch/3, Compare To Zero/1
  laneIn/1 -> Add/2
  Compare To Zero/1 -> Multiport Switch1/1, Multiport Switch/1

== system HDL_source/FPGALaneDetection/Lane Detection Algorithm/ComputeEgoLanes1/FirstPassEgoLane/Subsystem5 ==
  laneIn : Inport
  Frame_Center_PCIe : Inport  Port=2
  Abs1 : Abs
  Add : Sum  Inputs=+-  OutDataTypeStr=fixdt(1,12,0)
  Compare To Zero : simulink/Logic and Bit Operations/Compare To Zero  relop=<=  OutDataTypeStr=boolean
  Constant7 : Constant  Value=1000  OutDataTypeStr=fixdt(1,12,0)  SampleTime=-1
  Delay : Delay  DelayLength=1
  Delay1 : Delay  DelayLength=1
  Multiport Switch : MultiPortSwitch  DataPortOrder=Zero-based contiguous  Inputs=2  zeroidx=on
  Multiport Switch1 : MultiPortSwitch  DataPortOrder=Zero-based contiguous  Inputs=2  zeroidx=on
  RightLaneVal : Outport
  LeftLaneVal : Outport  Port=2
  wires:
  Compare To Zero/1 -> Multiport Switch/1, Multiport Switch1/1
  laneIn/1 -> Add/2
  Add/1 -> Compare To Zero/1, Multiport Switch/3, Multiport Switch1/2
  Multiport Switch/1 -> Abs1/1
  Constant7/1 -> Multiport Switch/2, Multiport Switch1/3
  Frame_Center_PCIe/1 -> Add/1
  Multiport Switch1/1 -> Delay1/1
  Abs1/1 -> Delay/1
  Delay/1 -> RightLaneVal/1
  Delay1/1 -> LeftLaneVal/1

== system HDL_source/FPGALaneDetection/Lane Detection Algorithm/ComputeEgoLanes1/FirstPassEgoLane/Subsystem6 ==
  laneIn : Inport
  Frame_Center_PCIe : Inport  Port=2
  Abs1 : Abs
  Add : Sum  Inputs=+-  OutDataTypeStr=fixdt(1,12,0)
  Compare To Zero : simulink/Logic and Bit Operations/Compare To Zero  relop=<=  OutDataTypeStr=boolean
  Constant7 : Constant  Value=1000  OutDataTypeStr=fixdt(1,12,0)  SampleTime=-1
  Delay : Delay  DelayLength=1
  Delay1 : Delay  DelayLength=1
  Multiport Switch : MultiPortSwitch  DataPortOrder=Zero-based contiguous  Inputs=2  zeroidx=on
  Multiport Switch1 : MultiPortSwitch  DataPortOrder=Zero-based contiguous  Inputs=2  zeroidx=on
  RightLaneVal : Outport
  LeftLaneVal : Outport  Port=2
  wires:
  Delay1/1 -> LeftLaneVal/1
  Delay/1 -> RightLaneVal/1
  Abs1/1 -> Delay/1
  Multiport Switch1/1 -> Delay1/1
  Frame_Center_PCIe/1 -> Add/1
  Constant7/1 -> Multiport Switch1/3, Multiport Switch/2
  Multiport Switch/1 -> Abs1/1
  Add/1 -> Multiport Switch1/2, Multiport Switch/3, Compare To Zero/1
  laneIn/1 -> Add/2
  Compare To Zero/1 -> Multiport Switch1/1, Multiport Switch/1

== system HDL_source/FPGALaneDetection/Lane Detection Algorithm/ComputeEgoLanes1/FirstPassEgoLane/Subsystem7 ==
  laneIn : Inport
  Frame_Center_PCIe : Inport  Port=2
  Abs1 : Abs
  Add : Sum  Inputs=+-  OutDataTypeStr=fixdt(1,12,0)
  Compare To Zero : simulink/Logic and Bit Operations/Compare To Zero  relop=<=  OutDataTypeStr=boolean
  Constant7 : Constant  Value=1000  OutDataTypeStr=fixdt(1,12,0)  SampleTime=-1
  Delay : Delay  DelayLength=1
  Delay1 : Delay  DelayLength=1
  Multiport Switch : MultiPortSwitch  DataPortOrder=Zero-based contiguous  Inputs=2  zeroidx=on
  Multiport Switch1 : MultiPortSwitch  DataPortOrder=Zero-based contiguous  Inputs=2  zeroidx=on
  RightLaneVal : Outport
  LeftLaneVal : Outport  Port=2
  wires:
  Compare To Zero/1 -> Multiport Switch/1, Multiport Switch1/1
  laneIn/1 -> Add/2
  Add/1 -> Compare To Zero/1, Multiport Switch/3, Multiport Switch1/2
  Multiport Switch/1 -> Abs1/1
  Constant7/1 -> Multiport Switch/2, Multiport Switch1/3
  Frame_Center_PCIe/1 -> Add/1
  Multiport Switch1/1 -> Delay1/1
  Abs1/1 -> Delay/1
  Delay/1 -> RightLaneVal/1
  Delay1/1 -> LeftLaneVal/1

== system HDL_source/FPGALaneDetection/Lane Detection Algorithm/ComputeEgoLanes1/FirstPassEgoLane/rightminop ==
  val1 : Inport
  val2 : Inport  Port=2
  ind1 : Inport  Port=3
  ind2 : Inport  Port=4
  Delay{,1..5} (6 alike) : Delay  DelayLength=1
  Multiport Switch : MultiPortSwitch  DataPortOrder=Zero-based contiguous  Inputs=2  zeroidx=on
  Multiport Switch1 : MultiPortSwitch  DataPortOrder=Zero-based contiguous  Inputs=2  zeroidx=on
  Relational Operator : RelationalOperator  Operator=<=  OutDataTypeStr=boolean  RndMeth=Simplest
  valmin : Outport
  indmin : Outport  Port=2
  wires:
  val1/1 -> Delay2/1
  Multiport Switch1/1 -> Delay1/1
  val2/1 -> Delay3/1
  ind1/1 -> Delay4/1
  Multiport Switch/1 -> Delay/1
  Relational Operator/1 -> Multiport Switch/1, Multiport Switch1/1
  ind2/1 -> Delay5/1
  Delay/1 -> valmin/1
  Delay1/1 -> indmin/1
  Delay2/1 -> Relational Operator/1, Multiport Switch/3
  Delay3/1 -> Relational Operator/2, Multiport Switch/2
  Delay4/1 -> Multiport Switch1/3
  Delay5/1 -> Multiport Switch1/2

== system HDL_source/FPGALaneDetection/Lane Detection Algorithm/ComputeEgoLanes1/FirstPassEgoLane/rightminop1 ==
  val1 : Inport
  val2 : Inport  Port=2
  ind1 : Inport  Port=3
  ind2 : Inport  Port=4
  Delay{,1..5} (6 alike) : Delay  DelayLength=1
  Multiport Switch : MultiPortSwitch  DataPortOrder=Zero-based contiguous  Inputs=2  zeroidx=on
  Multiport Switch1 : MultiPortSwitch  DataPortOrder=Zero-based contiguous  Inputs=2  zeroidx=on
  Relational Operator : RelationalOperator  Operator=<=  OutDataTypeStr=boolean  RndMeth=Simplest
  valmin : Outport
  indmin : Outport  Port=2
  wires:
  Delay5/1 -> Multiport Switch1/2
  Delay4/1 -> Multiport Switch1/3
  Delay3/1 -> Multiport Switch/2, Relational Operator/2
  Delay2/1 -> Multiport Switch/3, Relational Operator/1
  Delay1/1 -> indmin/1
  Delay/1 -> valmin/1
  ind2/1 -> Delay5/1
  Relational Operator/1 -> Multiport Switch1/1, Multiport Switch/1
  Multiport Switch/1 -> Delay/1
  ind1/1 -> Delay4/1
  val2/1 -> Delay3/1
  Multiport Switch1/1 -> Delay1/1
  val1/1 -> Delay2/1

== system HDL_source/FPGALaneDetection/Lane Detection Algorithm/ComputeEgoLanes1/FirstPassEgoLane/rightminop10 ==
  val1 : Inport
  val2 : Inport  Port=2
  ind1 : Inport  Port=3
  ind2 : Inport  Port=4
  Delay{,1..5} (6 alike) : Delay  DelayLength=1
  Multiport Switch : MultiPortSwitch  DataPortOrder=Zero-based contiguous  Inputs=2  zeroidx=on
  Multiport Switch1 : MultiPortSwitch  DataPortOrder=Zero-based contiguous  Inputs=2  zeroidx=on
  Relational Operator : RelationalOperator  Operator=<=  OutDataTypeStr=boolean  RndMeth=Simplest
  valmin : Outport
  indmin : Outport  Port=2
  wires:
  val1/1 -> Delay2/1
  Multiport Switch1/1 -> Delay1/1
  val2/1 -> Delay3/1
  ind1/1 -> Delay4/1
  Multiport Switch/1 -> Delay/1
  Relational Operator/1 -> Multiport Switch/1, Multiport Switch1/1
  ind2/1 -> Delay5/1
  Delay/1 -> valmin/1
  Delay1/1 -> indmin/1
  Delay2/1 -> Relational Operator/1, Multiport Switch/3
  Delay3/1 -> Relational Operator/2, Multiport Switch/2
  Delay4/1 -> Multiport Switch1/3
  Delay5/1 -> Multiport Switch1/2

== system HDL_source/FPGALaneDetection/Lane Detection Algorithm/ComputeEgoLanes1/FirstPassEgoLane/rightminop11 ==
  val1 : Inport
  val2 : Inport  Port=2
  ind1 : Inport  Port=3
  ind2 : Inport  Port=4
  Delay{,1..5} (6 alike) : Delay  DelayLength=1
  Multiport Switch : MultiPortSwitch  DataPortOrder=Zero-based contiguous  Inputs=2  zeroidx=on
  Multiport Switch1 : MultiPortSwitch  DataPortOrder=Zero-based contiguous  Inputs=2  zeroidx=on
  Relational Operator : RelationalOperator  Operator=<=  OutDataTypeStr=boolean  RndMeth=Simplest
  valmin : Outport
  indmin : Outport  Port=2
  wires:
  Delay5/1 -> Multiport Switch1/2
  Delay4/1 -> Multiport Switch1/3
  Delay3/1 -> Multiport Switch/2, Relational Operator/2
  Delay2/1 -> Multiport Switch/3, Relational Operator/1
  Delay1/1 -> indmin/1
  Delay/1 -> valmin/1
  ind2/1 -> Delay5/1
  Relational Operator/1 -> Multiport Switch1/1, Multiport Switch/1
  Multiport Switch/1 -> Delay/1
  ind1/1 -> Delay4/1
  val2/1 -> Delay3/1
  Multiport Switch1/1 -> Delay1/1
  val1/1 -> Delay2/1

== system HDL_source/FPGALaneDetection/Lane Detection Algorithm/ComputeEgoLanes1/FirstPassEgoLane/rightminop2 ==
  val1 : Inport
  val2 : Inport  Port=2
  ind1 : Inport  Port=3
  ind2 : Inport  Port=4
  Delay{,1..5} (6 alike) : Delay  DelayLength=1
  Multiport Switch : MultiPortSwitch  DataPortOrder=Zero-based contiguous  Inputs=2  zeroidx=on
  Multiport Switch1 : MultiPortSwitch  DataPortOrder=Zero-based contiguous  Inputs=2  zeroidx=on
  Relational Operator : RelationalOperator  Operator=<=  OutDataTypeStr=boolean  RndMeth=Simplest
  valmin : Outport
  indmin : Outport  Port=2
  wires:
  val1/1 -> Delay2/1
  Multiport Switch1/1 -> Delay1/1
  val2/1 -> Delay3/1
  ind1/1 -> Delay4/1
  Multiport Switch/1 -> Delay/1
  Relational Operator/1 -> Multiport Switch/1, Multiport Switch1/1
  ind2/1 -> Delay5/1
  Delay/1 -> valmin/1
  Delay1/1 -> indmin/1
  Delay2/1 -> Relational Operator/1, Multiport Switch/3
  Delay3/1 -> Relational Operator/2, Multiport Switch/2
  Delay4/1 -> Multiport Switch1/3
  Delay5/1 -> Multiport Switch1/2

== system HDL_source/FPGALaneDetection/Lane Detection Algorithm/ComputeEgoLanes1/FirstPassEgoLane/rightminop3 ==
  val1 : Inport
  val2 : Inport  Port=2
  ind1 : Inport  Port=3
  ind2 : Inport  Port=4
  Delay{,1..5} (6 alike) : Delay  DelayLength=1
  Multiport Switch : MultiPortSwitch  DataPortOrder=Zero-based contiguous  Inputs=2  zeroidx=on
  Multiport Switch1 : MultiPortSwitch  DataPortOrder=Zero-based contiguous  Inputs=2  zeroidx=on
  Relational Operator : RelationalOperator  Operator=<=  OutDataTypeStr=boolean  RndMeth=Simplest
  valmin : Outport
  indmin : Outport  Port=2
  wires:
  Delay5/1 -> Multiport Switch1/2
  Delay4/1 -> Multiport Switch1/3
  Delay3/1 -> Multiport Switch/2, Relational Operator/2
  Delay2/1 -> Multiport Switch/3, Relational Operator/1
  Delay1/1 -> indmin/1
  Delay/1 -> valmin/1
  ind2/1 -> Delay5/1
  Relational Operator/1 -> Multiport Switch1/1, Multiport Switch/1
  Multiport Switch/1 -> Delay/1
  ind1/1 -> Delay4/1
  val2/1 -> Delay3/1
  Multiport Switch1/1 -> Delay1/1
  val1/1 -> Delay2/1

== system HDL_source/FPGALaneDetection/Lane Detection Algorithm/ComputeEgoLanes1/FirstPassEgoLane/rightminop4 ==
  val1 : Inport
  val2 : Inport  Port=2
  ind1 : Inport  Port=3
  ind2 : Inport  Port=4
  Delay{,1..5} (6 alike) : Delay  DelayLength=1
  Multiport Switch : MultiPortSwitch  DataPortOrder=Zero-based contiguous  Inputs=2  zeroidx=on
  Multiport Switch1 : MultiPortSwitch  DataPortOrder=Zero-based contiguous  Inputs=2  zeroidx=on
  Relational Operator : RelationalOperator  Operator=<=  OutDataTypeStr=boolean  RndMeth=Simplest
  valmin : Outport
  indmin : Outport  Port=2
  wires:
  val1/1 -> Delay2/1
  Multiport Switch1/1 -> Delay1/1
  val2/1 -> Delay3/1
  ind1/1 -> Delay4/1
  Multiport Switch/1 -> Delay/1
  Relational Operator/1 -> Multiport Switch/1, Multiport Switch1/1
  ind2/1 -> Delay5/1
  Delay/1 -> valmin/1
  Delay1/1 -> indmin/1
  Delay2/1 -> Relational Operator/1, Multiport Switch/3
  Delay3/1 -> Relational Operator/2, Multiport Switch/2
  Delay4/1 -> Multiport Switch1/3
  Delay5/1 -> Multiport Switch1/2

== system HDL_source/FPGALaneDetection/Lane Detection Algorithm/ComputeEgoLanes1/FirstPassEgoLane/rightminop5 ==
  val1 : Inport
  val2 : Inport  Port=2
  ind1 : Inport  Port=3
  ind2 : Inport  Port=4
  Delay{,1..5} (6 alike) : Delay  DelayLength=1
  Multiport Switch : MultiPortSwitch  DataPortOrder=Zero-based contiguous  Inputs=2  zeroidx=on
  Multiport Switch1 : MultiPortSwitch  DataPortOrder=Zero-based contiguous  Inputs=2  zeroidx=on
  Relational Operator : RelationalOperator  Operator=<=  OutDataTypeStr=boolean  RndMeth=Simplest
  valmin : Outport
  indmin : Outport  Port=2
  wires:
  Delay5/1 -> Multiport Switch1/2
  Delay4/1 -> Multiport Switch1/3
  Delay3/1 -> Multiport Switch/2, Relational Operator/2
  Delay2/1 -> Multiport Switch/3, Relational Operator/1
  Delay1/1 -> indmin/1
  Delay/1 -> valmin/1
  ind2/1 -> Delay5/1
  Relational Operator/1 -> Multiport Switch1/1, Multiport Switch/1
  Multiport Switch/1 -> Delay/1
  ind1/1 -> Delay4/1
  val2/1 -> Delay3/1
  Multiport Switch1/1 -> Delay1/1
  val1/1 -> Delay2/1
